simulink model "etc_parent"  (R2018a)
settings: Solver=ode45  StartTime=0.0  StopTime=20.0  RelTol=1e-3
PreLoadFcn:
  | etc_all_data;
values from neighbouring files (symbols this model uses):
  degConv = 180/pi    (= 57.2957795131)    [etc_all_data.m]
undefined symbols (not defined in the file or in its folder): Cs, J, Kd, Ki, Kp, Ks, theta_eq, Ts
Description:
  | This is my help
settings Model: ParamWorkspaceSource=ReferencedWorkspace  Creator=nicholas  LastModifiedBy=bneiswan
settings DataIOCC: LimitDataPoints=on  SaveFormat=Array  SignalLoggingName=sigsOut
settings OptimizationCC: ExpressionDepthLimit=2147483647  InitFltsAndDblsToZero=on  LifeSpan=inf
settings DebuggingCC: SaveWithParameterizedLinksMsg=none  UnderspecifiedInitializationDetection=Classic  MergeDetectMultiDrivingBlocksExec=none  SignalResolutionControl=TryResolveAllWithWarning  MultiTaskDSMMsg=warning  MultiTaskCondExecSysMsg=none  ParameterPrecisionLossMsg=none  FcnCallInpInsideContextMsg=warning  AllowSymbolicDim=off  StateNameClashWarn=warning  SFUnexpectedBacktrackingDiag=warning  SFNoUnconditionalDefaultTransitionDiag=warning  SFExecutionAtInitializationDiag=none
settings HardwareCC: ProdBitPerPointer=32  ProdBitPerSizeT=32  ProdBitPerPtrDiffT=32  ProdLargestAtomicFloat=None  ProdIntDivRoundTo=Undefined  ProdEndianess=Unspecified  ProdWordSize=32  ProdHWDeviceType=32-bit Generic  TargetIntDivRoundTo=Zero  TargetEndianess=BigEndian  TargetHWDeviceType=Motorola PowerPC
settings ModelReferenceCC: PropagateSignalLabelsOutOfModel=off
settings SFSimCC: SimParseCustomCode=off
settings CodeAppCC: StateflowObjectComments=on
settings GRTTargetCC: TargetFcnLib=ansi_tfl_tmw.mat  TargetLangStandard=C89/C90 (ANSI)  GeneratePreprocessorConditionals=Disable all  CombineOutputUpdateFcns=off  GRTInterface=on
settings ConfigComp: CovMetricSettings=dw  CovHtmlReporting=on  CovSaveCumulativeToWorkspaceVar=on  CovSaveSingleToWorkspaceVar=on  CovExternalEMLEnable=off  CovSFcnEnable=off

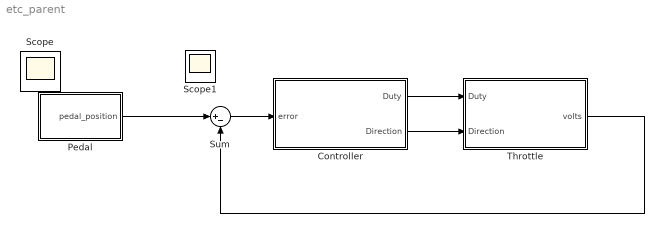
== system etc_parent ==
  Controller : Subsystem
  Pedal : Subsystem
  Sum : Sum  Inputs=|+-
  Throttle : Subsystem
  Scope : Scope
  Scope1 : Scope
  wires:
  Controller/1(Duty) -> Throttle/1(Duty)
  Controller/2(Direction) -> Throttle/2(Direction)
  Pedal/1(pedal_position) -> Sum/1
  Sum/1 -> Controller/1(error)
  Throttle/1(volts) -> Sum/2

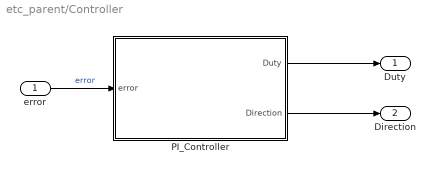
== system etc_parent/Controller ==
  error : Inport
  PI_Controller : Subsystem
  Duty : Outport
  Direction : Outport  Port=2
  wires:
  PI_Controller/2(Direction) -> Direction/1
  PI_Controller/1(Duty) -> Duty/1
  error/1 -> PI_Controller/1(error)  "error"

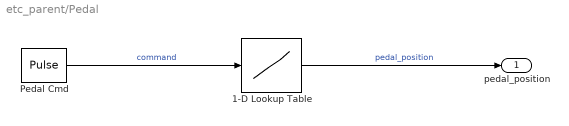
== system etc_parent/Pedal ==
  1-D Lookup Table : Lookup_n-D  NumberOfTableDimensions=1  BreakpointsForDimension1=[0 1]  Table=[0.5 4.5]  RndMeth=Simplest  InputSameDT=on
  Pedal Cmd : DiscretePulseGenerator  PulseType=Time based  Amplitude=0.9  Period=10  PulseWidth=50  PhaseDelay=2.5
  pedal_position : Outport
  wires:
  Pedal Cmd/1 -> 1-D Lookup Table/1  "command"
  1-D Lookup Table/1 -> pedal_position/1  "pedal_position"

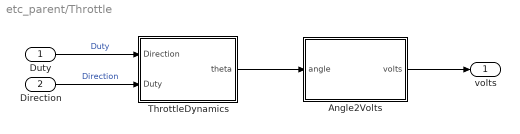
== system etc_parent/Throttle ==
  Duty : Inport
  Direction : Inport  Port=2
  Angle2Volts : Subsystem
  ThrottleDynamics : Subsystem
  volts : Outport
  wires:
  ThrottleDynamics/1(theta) -> Angle2Volts/1("angle ")
  Angle2Volts/1(volts) -> volts/1
  Duty/1 -> ThrottleDynamics/1(Direction)  "Duty"
  Direction/1 -> ThrottleDynamics/2(Duty)  "Direction"

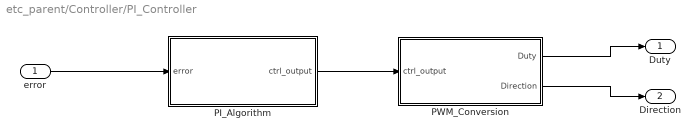
== system etc_parent/Controller/PI_Controller ==
  error : Inport  SampleTime=Ts
  PI_Algorithm : Subsystem
  PWM_Conversion : Subsystem
  Duty : Outport
  Direction : Outport  Port=2
  wires:
  PI_Algorithm/1(ctrl_output) -> PWM_Conversion/1(ctrl_output)
  PWM_Conversion/2(Direction) -> Direction/1
  PWM_Conversion/1("Duty ") -> Duty/1
  error/1 -> PI_Algorithm/1(error)

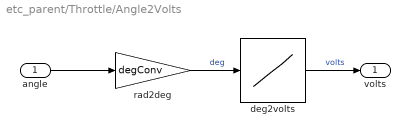
== system etc_parent/Throttle/Angle2Volts ==
  "angle " : Inport
  deg2volts : Lookup_n-D  NumberOfTableDimensions=1  BreakpointsForDimension1=[0 90]  Table=[0.5 4.5]  RndMeth=Simplest  InputSameDT=on
  rad2deg : Gain  Gain=degConv  SaturateOnIntegerOverflow=on  OutDataTypeStr=Inherit: Same as input  ParamDataTypeStr=Inherit: Same as input
  volts : Outport
  wires:
  rad2deg/1 -> deg2volts/1  "deg"
  deg2volts/1 -> volts/1  "volts"
  "angle "/1 -> rad2deg/1

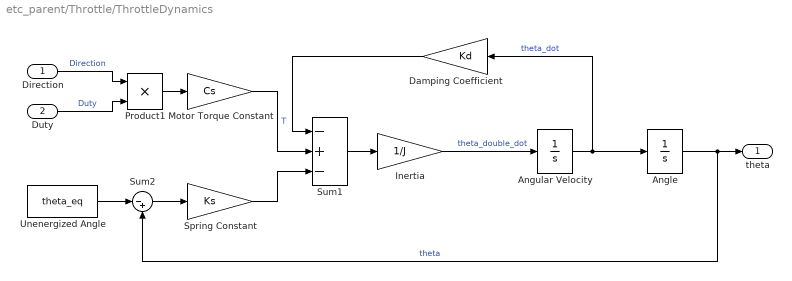
== system etc_parent/Throttle/ThrottleDynamics ==
  Direction : Inport
  Duty : Inport  Port=2
  Angle : Integrator  InitialCondition=pi/6  LimitOutput=on  UpperSaturationLimit=pi/2  LowerSaturationLimit=0
      settings: AttributesFormatString=Initial condition: %<InitialCondition>\n%<LowerSaturationLimit> <= theta <= %<UpperSaturationLimit>
  Angular Velocity : Integrator
      settings: AttributesFormatString=Initial condition: %<InitialCondition>
  Damping Coefficient : Gain  Gain=Kd  SaturateOnIntegerOverflow=on  OutDataTypeStr=Inherit: Same as input  ParamDataTypeStr=Inherit: Same as input
  Inertia : Gain  Gain=1/J  SaturateOnIntegerOverflow=on  OutDataTypeStr=Inherit: Same as input  ParamDataTypeStr=Inherit: Same as input
  Motor Torque Constant : Gain  Gain=Cs  SaturateOnIntegerOverflow=on  OutDataTypeStr=Inherit: Same as input  ParamDataTypeStr=Inherit: Same as input
  Product1 : Product  SaturateOnIntegerOverflow=on  OutDataTypeStr=Inherit: Same as first input
  Spring Constant : Gain  Gain=Ks  SaturateOnIntegerOverflow=on  OutDataTypeStr=Inherit: Same as input  ParamDataTypeStr=Inherit: Same as input
  Sum1 : Sum  Inputs=-+-  SaturateOnIntegerOverflow=on
  Sum2 : Sum  Inputs=|-+  SaturateOnIntegerOverflow=on
  Unenergized Angle : Constant  Value=theta_eq
  theta : Outport
  wires:
  Product1/1 -> Motor Torque Constant/1
  Unenergized Angle/1 -> Sum2/1
  Sum2/1 -> Spring Constant/1
  Angle/1 -> theta/1, Sum2/2  "theta"
  Angular Velocity/1 -> Angle/1, Damping Coefficient/1  "theta_dot"
  Inertia/1 -> Angular Velocity/1  "theta_double_dot"
  Sum1/1 -> Inertia/1
  Direction/1 -> Product1/1  "Direction"
  Duty/1 -> Product1/2  "Duty"
  Motor Torque Constant/1 -> Sum1/2  "T"
  Damping Coefficient/1 -> Sum1/1
  Spring Constant/1 -> Sum1/3

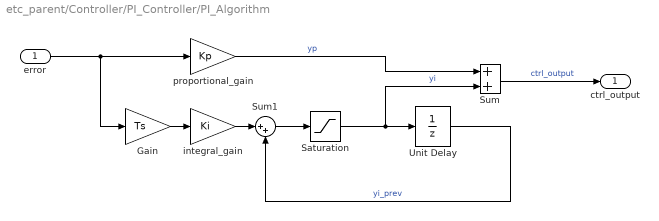
== system etc_parent/Controller/PI_Controller/PI_Algorithm ==
  error : Inport  SampleTime=Ts
      settings: AttributesFormatString=Sample time = %<SampleTime>
  Gain : Gain  Gain=Ts  SaturateOnIntegerOverflow=on  OutDataTypeStr=Inherit: Same as input  ParamDataTypeStr=Inherit: Same as input
  Saturation : Saturate  UpperLimit=1  LowerLimit=-1
      settings: AttributesFormatString=Max: %<UpperLimit>\nMin: %<LowerLimit>
  Sum : Sum  SaturateOnIntegerOverflow=on  InputSameDT=on  OutDataTypeStr=Inherit: Same as first input
  Sum1 : Sum  Inputs=|++  SaturateOnIntegerOverflow=on  InputSameDT=on  OutDataTypeStr=Inherit: Same as first input
  Unit Delay : UnitDelay  SampleTime=Ts
      settings: AttributesFormatString=yi0 = %<X0>\nSample time = %<SampleTime>
  integral_gain : Gain  Gain=Ki  SaturateOnIntegerOverflow=on  OutDataTypeStr=Inherit: Same as input  ParamDataTypeStr=Inherit: Same as input
  proportional_gain : Gain  Gain=Kp  SaturateOnIntegerOverflow=on  OutDataTypeStr=Inherit: Same as input  ParamDataTypeStr=Inherit: Same as input
  ctrl_output : Outport
  wires:
  Sum/1 -> ctrl_output/1  "ctrl_output"
  error/1 -> Gain/1, proportional_gain/1
  Saturation/1 -> Sum/2, Unit Delay/1  "yi"
  Sum1/1 -> Saturation/1
  Unit Delay/1 -> Sum1/2  "yi_prev"
  Gain/1 -> integral_gain/1
  integral_gain/1 -> Sum1/1
  proportional_gain/1 -> Sum/1  "yp"

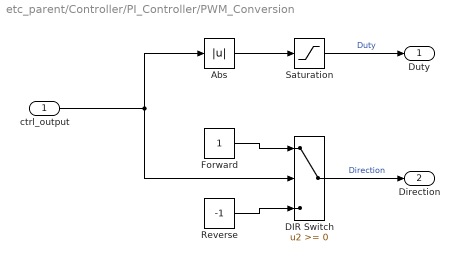
== system etc_parent/Controller/PI_Controller/PWM_Conversion ==
  ctrl_output : Inport
  Abs : Abs
  DIR Switch : Switch
      settings: AttributesFormatString=Criteria: %<Criteria>\nThreshold: %<Threshold>
  Forward : Constant  OutDataTypeStr=double
  Reverse : Constant  Value=-1  OutDataTypeStr=double
  Saturation : Saturate  UpperLimit=1  LowerLimit=0
      settings: AttributesFormatString=%<LowerLimit> < duty < %<UpperLimit>
  "Duty " : Outport
  Direction : Outport  Port=2
  wires:
  ctrl_output/1 -> Abs/1, DIR Switch/2
  Forward/1 -> DIR Switch/1
  Reverse/1 -> DIR Switch/3
  DIR Switch/1 -> Direction/1  "Direction"
  Saturation/1 -> "Duty "/1  "Duty"
  Abs/1 -> Saturation/1
